simulink library "Kitchen_Lib"  (R2023a)
settings: Solver=VariableStepAuto  StartTime=0.0  StopTime=10.0  RelTol=1e-3  EnableMultiTasking=on
undefined symbols (not defined in the file): Kitc_BusTyp_P, Kitc_BusTypSkyr_C, Kitc_ColrLedColrls_C, Kitc_ColrLedGrn_C, Kitc_ColrLedRed_C, Kitc_ColrLedYlw_C, Kitc_StDgnWtrTank_C, Kitc_StElecPlugScktOffByClmp50_P, Kitc_StsDlyBlink_C, Kitc_StsErrBlink_C, Kitc_StsFctAcvn_P, Kitc_StsInfoBlink_C, Kitc_StsKitchnOffAutoIgOff_P, Kitc_StsKitchnOffBySwt_P, Kitc_StsKitchnOffDoorLockd_P, Kitc_StsKitchnOffIgOff_P, Kitc_StsKitchnOffUv_P, Kitc_StsKitchnOnBySwt_P, Kitc_StsKitchnOnNVM_P, Kitc_StsLedOff_C, Kitc_StsLedOn_C, Kitc_StsLrgCnsAcv_P, Kitc_StTrfrAnSwtInstd_P, Kitc_StTrfrSwtInstd_P, Kitc_TiKitcRefgtrOffDly_P, Kitc_ULowrThdBat_C, Kitc_UUpprThdBat_C, Kitc_ValFalse_C, Kitc_ValPwmFreq2_C, Kitc_ValPwmFreq_C, Kitc_ValTrue_C
libraries: MAN_Library x50, E2E_Lib x3
(part 2 of 13)

== system Kitchen_Lib/Kitchen/100ms/Kitchn/Subsystem1/Subsystem1 ==
  Kitc_StsHostsCallAcv : Inport
  BOOLEAN_TO_UINT8_Signals : Subsystem  AncestorBlock=E2E_Lib/BOOLEAN_TO_UINT8_Signals
  Logical Operator1 : Logic  Operator=NOT  AllPortsSameDT=off  OutDataTypeStr=boolean
  LogicalOperator25 : Logic  AllPortsSameDT=off  OutDataTypeStr=boolean
  Terminator : Terminator
  Terminator1 : Terminator
  Kitc_StsHostsCallAcv_E2E : Outport
  wires:
  Logical Operator1/1 -> LogicalOperator25/1
  BOOLEAN_TO_UINT8_Signals/3(Error) -> Terminator/1
  BOOLEAN_TO_UINT8_Signals/1(SignalOff) -> Logical Operator1/1
  BOOLEAN_TO_UINT8_Signals/4(NotInstalled_NotAvailable) -> Terminator1/1
  Kitc_StsHostsCallAcv/1 -> BOOLEAN_TO_UINT8_Signals/1(BOOLEAN_TO_UINT8_SignalIn)
  BOOLEAN_TO_UINT8_Signals/2(Signal|On) -> LogicalOperator25/2
  LogicalOperator25/1 -> Kitc_StsHostsCallAcv_E2E/1

== system Kitchen_Lib/Kitchen/100ms/Kitchn/Subsystem1/Subsystem10 ==
  GW_W_output : Inport
  Terminator40 : Terminator
  Terminator41 : Terminator
  UINT8_Signal : Subsystem  AncestorBlock=E2E_Lib/UINT8_Signal
  wires:
  UINT8_Signal/1(Error) -> Terminator40/1
  GW_W_output/1 -> UINT8_Signal/1(UINT8_SignalIn)
  UINT8_Signal/2(NotInstalled_NotAvailable) -> Terminator41/1

== system Kitchen_Lib/Kitchen/100ms/Kitchn/Subsystem1/Subsystem11 ==
  GW_BusTyp : Inport
  Terminator40 : Terminator
  Terminator41 : Terminator
  UINT8_Signal : Subsystem  AncestorBlock=E2E_Lib/UINT8_Signal
  wires:
  UINT8_Signal/2(NotInstalled_NotAvailable) -> Terminator41/1
  GW_BusTyp/1 -> UINT8_Signal/1(UINT8_SignalIn)
  UINT8_Signal/1(Error) -> Terminator40/1

== system Kitchen_Lib/Kitchen/100ms/Kitchn/Subsystem1/Subsystem12 ==
  GW_SpdGrtr3 : Inport
  BOOLEAN_TO_UINT8_Signals : Subsystem  AncestorBlock=E2E_Lib/BOOLEAN_TO_UINT8_Signals
  Logical Operator : Logic  AllPortsSameDT=off  OutDataTypeStr=boolean
  Logical Operator1 : Logic  Operator=NOT  AllPortsSameDT=off  OutDataTypeStr=boolean
  Terminator : Terminator
  Terminator1 : Terminator
  GW_SpdGrtr3_E2E : Outport
  wires:
  BOOLEAN_TO_UINT8_Signals/2(Signal|On) -> Logical Operator/2
  BOOLEAN_TO_UINT8_Signals/4(NotInstalled_NotAvailable) -> Terminator1/1
  BOOLEAN_TO_UINT8_Signals/3(Error) -> Terminator/1
  Logical Operator1/1 -> Logical Operator/1
  GW_SpdGrtr3/1 -> BOOLEAN_TO_UINT8_Signals/1(BOOLEAN_TO_UINT8_SignalIn)
  Logical Operator/1 -> GW_SpdGrtr3_E2E/1
  BOOLEAN_TO_UINT8_Signals/1(SignalOff) -> Logical Operator1/1

== system Kitchen_Lib/Kitchen/100ms/Kitchn/Subsystem1/Subsystem13 ==
  DBF_StsDoor1Open : Inport
  BOOLEAN_TO_UINT8_Signals : Subsystem  AncestorBlock=E2E_Lib/BOOLEAN_TO_UINT8_Signals
  Logical Operator1 : Logic  Operator=NOT  AllPortsSameDT=off  OutDataTypeStr=boolean
  LogicalOperator25 : Logic  AllPortsSameDT=off  OutDataTypeStr=boolean
  Terminator : Terminator
  Terminator1 : Terminator
  DBF_StsDoor1Open_E2E : Outport
  wires:
  BOOLEAN_TO_UINT8_Signals/3(Error) -> Terminator/1
  BOOLEAN_TO_UINT8_Signals/1(SignalOff) -> Logical Operator1/1
  BOOLEAN_TO_UINT8_Signals/4(NotInstalled_NotAvailable) -> Terminator1/1
  DBF_StsDoor1Open/1 -> BOOLEAN_TO_UINT8_Signals/1(BOOLEAN_TO_UINT8_SignalIn)
  BOOLEAN_TO_UINT8_Signals/2(Signal|On) -> LogicalOperator25/2
  LogicalOperator25/1 -> DBF_StsDoor1Open_E2E/1
  Logical Operator1/1 -> LogicalOperator25/1

== system Kitchen_Lib/Kitchen/100ms/Kitchn/Subsystem1/Subsystem14 ==
  Toi_ToiInstlldInfo : Inport
  BOOLEAN_TO_UINT8_Signals : Subsystem  AncestorBlock=E2E_Lib/BOOLEAN_TO_UINT8_Signals
  Logical Operator1 : Logic  Operator=NOT  AllPortsSameDT=off  OutDataTypeStr=boolean
  LogicalOperator25 : Logic  AllPortsSameDT=off  OutDataTypeStr=boolean
  Terminator : Terminator
  Terminator1 : Terminator
  Toi_ToiInstlldInfo_E2E : Outport
  wires:
  Logical Operator1/1 -> LogicalOperator25/1
  LogicalOperator25/1 -> Toi_ToiInstlldInfo_E2E/1
  BOOLEAN_TO_UINT8_Signals/2(Signal|On) -> LogicalOperator25/2
  Toi_ToiInstlldInfo/1 -> BOOLEAN_TO_UINT8_Signals/1(BOOLEAN_TO_UINT8_SignalIn)
  BOOLEAN_TO_UINT8_Signals/4(NotInstalled_NotAvailable) -> Terminator1/1
  BOOLEAN_TO_UINT8_Signals/1(SignalOff) -> Logical Operator1/1
  BOOLEAN_TO_UINT8_Signals/3(Error) -> Terminator/1

== system Kitchen_Lib/Kitchen/100ms/Kitchn/Subsystem1/Subsystem15 ==
  Kitc_StDemoBd : Inport
  BOOLEAN_TO_UINT8_Signals : Subsystem  AncestorBlock=E2E_Lib/BOOLEAN_TO_UINT8_Signals
  Logical Operator1 : Logic  Operator=NOT  AllPortsSameDT=off  OutDataTypeStr=boolean
  LogicalOperator25 : Logic  AllPortsSameDT=off  OutDataTypeStr=boolean
  Terminator : Terminator
  Terminator1 : Terminator
  Kitc_StDemoBd_E2E : Outport
  wires:
  Logical Operator1/1 -> LogicalOperator25/1
  BOOLEAN_TO_UINT8_Signals/3(Error) -> Terminator/1
  BOOLEAN_TO_UINT8_Signals/1(SignalOff) -> Logical Operator1/1
  BOOLEAN_TO_UINT8_Signals/4(NotInstalled_NotAvailable) -> Terminator1/1
  Kitc_StDemoBd/1 -> BOOLEAN_TO_UINT8_Signals/1(BOOLEAN_TO_UINT8_SignalIn)
  BOOLEAN_TO_UINT8_Signals/2(Signal|On) -> LogicalOperator25/2
  LogicalOperator25/1 -> Kitc_StDemoBd_E2E/1

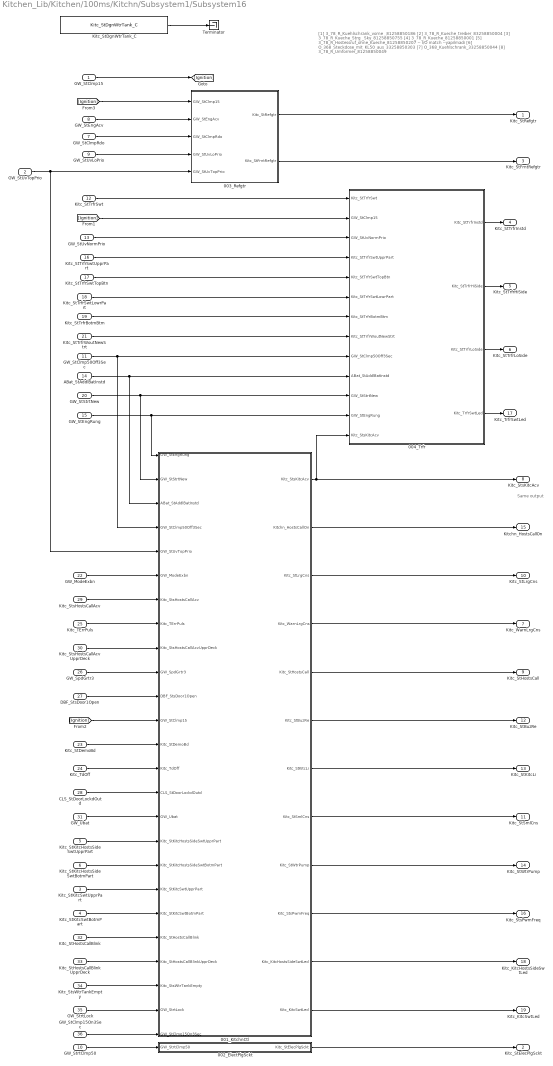
== system Kitchen_Lib/Kitchen/100ms/Kitchn/Subsystem1/Subsystem16 ==
  note: Same output
  note: [1] 3_78_R_Kuehlschrank_vorne _81258850186
      | [2] 3_78_R_Kueche_treiber_83258850004
      | [3] 3_78_R_Kueche_Strg _Sky_81258850755
      | [4] 3_78_R_Kueche_81258850001
      | [5] 3_78_R_Hostessruf_ohne_Kueche_81258850207 -- I/O match --yapilmadi
      | [6] O_368_Steckdose_mit_KL50_aus_33258850303
      | [7] O_368_Kuehlschrank_33258850044
      | [8] 3_78_R_Umformer_81258850049
  GW_StClmp15 : Inport
  "GW_StUvTopPrio " : Inport  Port=2
  Kitc_StKitcSwtUpprPart : Inport  Port=3
  Kitc_StKitcSwtBotmPart : Inport  Port=4
  Kitc_StKitcHostsSideSwtUpprPart : Inport  Port=5
  Kitc_StKitcHostsSideSwtBotmPart : Inport  Port=6
  GW_StClmpRdo : Inport  Port=7
  "GW_StEngAcv " : Inport  Port=8
  "GW_StUvLoPrio " : Inport  Port=9
  "GW_StrtClmp50 " : Inport  Port=10
  "GW_StClmp50Off3Sec " : Inport  Port=11
  "Kitc_StTrfrSwt " : Inport  Port=12
  "GW_StUvNormPrio " : Inport  Port=13
  ABat_StAddlBatInstd : Inport  Port=14
  GW_StEngRung : Inport  Port=15
  Kitc_StTrfrSwtUpprPart : Inport  Port=16
  Kitc_StTrfrSwtTopBtn : Inport  Port=17
  Kitc_StTrfrSwtLowrPart : Inport  Port=18
  Kitc_StTrfrBotmBtm : Inport  Port=19
  "GW_StStrtNew " : Inport  Port=20
  Kitc_StTrfrWoutNewStrt : Inport  Port=21
  "GW_ModeExbn " : Inport  Port=22
  Kitc_StDemoBd : Inport  Port=23
  Kitc_TdOff : Inport  Port=24
  Kitc_TErrPuls : Inport  Port=25
  GW_SpdGrtr3 : Inport  Port=26
  DBF_StsDoor1Open : Inport  Port=27
  CLS_StDoorLockdOutd : Inport  Port=28
  Kitc_StsHostsCallAcv : Inport  Port=29
  Kitc_StsHostsCallAcvUpprDeck : Inport  Port=30
  "GW_Ubat " : Inport  Port=31
  Kitc_StHostsCallBlink : Inport  Port=32
  Kitc_StHostsCallBlinkUpprDeck : Inport  Port=33
  Kitc_StsWtrTankEmpty : Inport  Port=34
  "GW_StrtLock " : Inport  Port=35
  "GW_StClmp15On3Sec " : Inport  Port=36
  001_KitchnCtl : Subsystem
  002_ElectPlgSckt : Subsystem
  003_Refgtr : Subsystem
  004_Trfr : Subsystem
  Kitc_StDgnWtrTank_C : Constant  Value=Kitc_StDgnWtrTank_C
  Terminator : Terminator
  Kitc_StRefgtr : Outport
  Kitc_StElecPlgSckt : Outport  Port=2
  Kitc_StFrntRefgtr : Outport  Port=3
  Kitc_StTrfrInstd : Outport  Port=4
  Kitc_StTrfrHiSide : Outport  Port=5
  Kitc_StTrfrLoSide : Outport  Port=6
  Kitc_WarnLrgCns : Outport  Port=7
  Kitc_StsKitcAcv : Outport  Port=8
  Kitc_StHostsCall : Outport  Port=9
  Kitc_StLrgCns : Outport  Port=10
  Kitc_StSmlCns : Outport  Port=11
  Kitc_StBuzRe : Outport  Port=12
  Kitc_StKitcLi : Outport  Port=13
  Kitc_StWtrPump : Outport  Port=14
  Kitchn_HostsCallOn : Outport  Port=15
  Kitc_StsPwmFreq : Outport  Port=16
  Kitc_TrfrSwtLed : Outport  Port=17
  Kitc_KitcHostsSideSwtLed : Outport  Port=18
  Kitc_KitcSwtLed : Outport  Port=19
  wires:
  "GW_StUvTopPrio "/1 -> 001_KitchnCtl/5("GW_StUvTopPrio "), 003_Refgtr/5("GW_StUvTopPrio ")
  Kitc_StKitcSwtUpprPart/1 -> 001_KitchnCtl/19(Kitc_StKitcSwtUpprPart)
  "GW_StEngAcv "/1 -> 003_Refgtr/2("GW_StEngAcv ")
  Kitc_StKitcSwtBotmPart/1 -> 001_KitchnCtl/20(Kitc_StKitcSwtBotmPart)
  "Kitc_StTrfrSwt "/1 -> 004_Trfr/1("Kitc_StTrfrSwt ")
  "GW_StClmp50Off3Sec "/1 -> 001_KitchnCtl/4("GW_StClmp50Off3Sec "), 004_Trfr/9("GW_StClmp50Off3Sec ")
  001_KitchnCtl/1(Kitc_StsKitcAcv) -> 004_Trfr/13(Kitc_StsKitcAcv), Kitc_StsKitcAcv/1
  "GW_StUvNormPrio "/1 -> 004_Trfr/3("GW_StUvNormPrio ")
  Kitc_StKitcHostsSideSwtBotmPart/1 -> 001_KitchnCtl/18(Kitc_StKitcHostsSideSwtBotmPart)
  "GW_StUvLoPrio "/1 -> 003_Refgtr/4("GW_StUvLoPrio ")
  "GW_StrtClmp50 "/1 -> 002_ElectPlgSckt/1("GW_StrtClmp50 ")
  Kitc_StKitcHostsSideSwtUpprPart/1 -> 001_KitchnCtl/17(Kitc_StKitcHostsSideSwtUpprPart)
  [Ignition] -> 003_Refgtr/1(GW_StClmp15)
  GW_StClmpRdo/1 -> 003_Refgtr/3(GW_StClmpRdo)
  Kitc_StsHostsCallAcv/1 -> 001_KitchnCtl/7(Kitc_StsHostsCallAcv)
  ABat_StAddlBatInstd/1 -> 001_KitchnCtl/3(ABat_StAddlBatInstd), 004_Trfr/10(ABat_StAddlBatInstd)
  Kitc_StTrfrSwtUpprPart/1 -> 004_Trfr/4(Kitc_StTrfrSwtUpprPart)
  GW_StClmp15/1 -> [Ignition]
  GW_StEngRung/1 -> 001_KitchnCtl/1(GW_StEngRung), 004_Trfr/12(GW_StEngRung)
  Kitc_TdOff/1 -> 001_KitchnCtl/14(Kitc_TdOff)
  Kitc_TErrPuls/1 -> 001_KitchnCtl/8(Kitc_TErrPuls)
  Kitc_StsHostsCallAcvUpprDeck/1 -> 001_KitchnCtl/9(Kitc_StsHostsCallAcvUpprDeck)
  Kitc_StTrfrSwtTopBtn/1 -> 004_Trfr/5(Kitc_StTrfrSwtTopBtn)
  "GW_StStrtNew "/1 -> 001_KitchnCtl/2("GW_StStrtNew "), 004_Trfr/11("GW_StStrtNew ")
  "GW_ModeExbn "/1 -> 001_KitchnCtl/6("GW_ModeExbn ")
  [Ignition] -> 004_Trfr/2(GW_StClmp15)
  [Ignition] -> 001_KitchnCtl/12(GW_StClmp15)
  GW_SpdGrtr3/1 -> 001_KitchnCtl/10(GW_SpdGrtr3)
  Kitc_StTrfrWoutNewStrt/1 -> 004_Trfr/8(Kitc_StTrfrWoutNewStrt)
  Kitc_StTrfrSwtLowrPart/1 -> 004_Trfr/6(Kitc_StTrfrSwtLowrPart)
  Kitc_StDemoBd/1 -> 001_KitchnCtl/13(Kitc_StDemoBd)
  CLS_StDoorLockdOutd/1 -> 001_KitchnCtl/15(CLS_StDoorLockdOutd)
  DBF_StsDoor1Open/1 -> 001_KitchnCtl/11(DBF_StsDoor1Open)
  Kitc_StTrfrBotmBtm/1 -> 004_Trfr/7(Kitc_StTrfrBotmBtm)
  "GW_Ubat "/1 -> 001_KitchnCtl/16("GW_Ubat ")
  Kitc_StsWtrTankEmpty/1 -> 001_KitchnCtl/23(Kitc_StsWtrTankEmpty)
  Kitc_StHostsCallBlink/1 -> 001_KitchnCtl/21(Kitc_StHostsCallBlink)
  "GW_StClmp15On3Sec "/1 -> 001_KitchnCtl/25("GW_StClmp15On3Sec ")
  "GW_StrtLock "/1 -> 001_KitchnCtl/24("GW_StrtLock ")
  Kitc_StHostsCallBlinkUpprDeck/1 -> 001_KitchnCtl/22(Kitc_StHostsCallBlinkUpprDeck)
  002_ElectPlgSckt/1(Kitc_StElecPlgSckt) -> Kitc_StElecPlgSckt/1
  001_KitchnCtl/8(Kitc_StSmlCns) -> Kitc_StSmlCns/1
  001_KitchnCtl/7(Kitc_StKitcLi) -> Kitc_StKitcLi/1
  001_KitchnCtl/6(Kitc_StBuzRe) -> Kitc_StBuzRe/1
  001_KitchnCtl/5(Kitc_StHostsCall) -> Kitc_StHostsCall/1
  001_KitchnCtl/4(Kitc_WarnLrgCns) -> Kitc_WarnLrgCns/1
  001_KitchnCtl/3(Kitc_StLrgCns) -> Kitc_StLrgCns/1
  004_Trfr/3(Kitc_StTrfrLoSide) -> Kitc_StTrfrLoSide/1
  004_Trfr/2(Kitc_StTrfrHiSide) -> Kitc_StTrfrHiSide/1
  004_Trfr/1(Kitc_StTrfrInstd) -> Kitc_StTrfrInstd/1
  003_Refgtr/2("Kitc_StFrntRefgtr ") -> Kitc_StFrntRefgtr/1
  003_Refgtr/1(Kitc_StRefgtr) -> Kitc_StRefgtr/1
  001_KitchnCtl/9(Kitc_StWtrPump) -> Kitc_StWtrPump/1
  001_KitchnCtl/2(Kitchn_HostsCallOn) -> Kitchn_HostsCallOn/1
  001_KitchnCtl/10(Kitc_StsPwmFreq) -> Kitc_StsPwmFreq/1
  Kitc_StDgnWtrTank_C/1 -> Terminator/1
  004_Trfr/4(Kitc_TrfrSwtLed) -> Kitc_TrfrSwtLed/1
  001_KitchnCtl/11(Kitc_KitcHostsSideSwtLed) -> Kitc_KitcHostsSideSwtLed/1
  001_KitchnCtl/12(Kitc_KitcSwtLed) -> Kitc_KitcSwtLed/1

== system Kitchen_Lib/Kitchen/100ms/Kitchn/Subsystem1/Subsystem17 ==
  Kitc_TdOff_E2E : Inport
  Terminator40 : Terminator
  Terminator41 : Terminator
  UINT32_Signal : Subsystem  AncestorBlock=E2E_Lib/UINT32_Signal
  wires:
  UINT32_Signal/1(Error) -> Terminator40/1
  UINT32_Signal/2(NotInstalled_NotAvailable) -> Terminator41/1
  Kitc_TdOff_E2E/1 -> UINT32_Signal/1(UINT32_SignalIn)

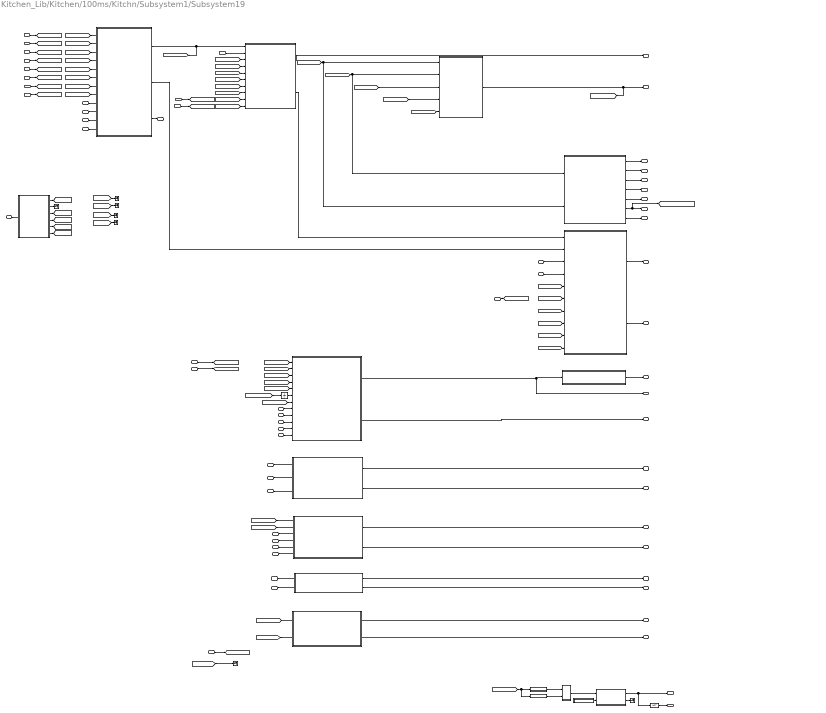
== system Kitchen_Lib/Kitchen/100ms/Kitchn/Subsystem1/Subsystem19 ==
  note: APPLICATION LOGIC
  note: OUTPUTS
  note: Skyliner
  note: EIO_B26 1Pin5
      | DigOut
      |
      | Kitc_StBuzRe
      | The pin of the call bell is given as a socket.
      | It is not connected to a serial or SA location on the device
      |
      | EIO_B26 4Pin22
      | DigOut
      | Kitc_StsKitcAcv
      | Kitchen activation signal.
      |
      | EIO_B26 1Pin2
      | PWMOut
      |
      | Kitc_StLrgCns
      |
      | It is the trigger pin that serves to activate the kitchen. When the button located in the fap section is pressed, the kitchen system is activated, and these pins are the trigger pins.
      |
      | EIO_B26 5Pin6
      | PWMOut
      |
      | Kitc_StSmlCns
      | There are two mode.
      | -When car is moving Large consumption mode is activated.
      | -When car is stopping Small consumption mode is activated.
      |
      | EIO_B26 5Pin7
      | DigOut
      |
      | Kitc_StTrfr
      | Kitchen power supply electrical plag.
      |
      | EIO_B26 3Pin2
      | DigInp
      |
      | Kitc_EidWtrTankEmpty
      | It reports the water level in the tank and sends a warning to the driver when the water runs out in the clean water
      |
      | EIO_B26 1Pin8
      | DigOut
      |
      | Kitc_StRefgtr
      | It is used for the refrigerator in cases where the refrigerator comes in the toilet
      |
      | EIO_B26 3Pin41
      | PWMOut
      | Kitc_StHostsCall
      | It is used for the hostess call Skyliner
  note: Shutdown Request
  Kitc_StKitcSwtUpprPart : Inport
  Kitc_StKitcHostsSideSwtUpprPart : Inport  Port=2
  Kitc_StKitcHostsSideSwtBotmPart : Inport  Port=3
  GW_StBttrySupplyVltMVBSWOn : Inport  Port=4
  "GW_ModeExbn " : Inport  Port=5
  GW_SpdGrtr3 : Inport  Port=6
  CLS_StDoorLockdOutd : Inport  Port=7
  "GW_StStrtNew " : Inport  Port=8
  GW_StUvTopPrio : Inport  Port=9
  GW_StClmp15 : Inport  Port=10
  DBF_StsDoor1Open : Inport  Port=11
  GW_StEngRung : Inport  Port=12
  ABat_StAddlBatInstd : Inport  Port=13
  Kitc_StsHostsCallAcv : Inport  Port=14
  "GW_StClmp50Off3Sec " : Inport  Port=15
  "GW_StUvNormPrio " : Inport  Port=16
  Kitc_StHostsCallBlink : Inport  Port=17
  Kitc_StHostsCallBlinkUpprDeck : Inport  Port=18
  Kitc_StsWtrTankEmpty : Inport  Port=19
  "GW_StrtLock " : Inport  Port=20
  "GW_StClmp15On3Sec " : Inport  Port=21
  Kitc_StsHostsCallAcvUpprDeck : Inport  Port=22
  Kitc_TErrPuls : Inport  Port=23
  Kitc_StTrfrSwtUpprPart : Inport  Port=24
  Kitc_StTrfrSwtTopBtn : Inport  Port=25
  Kitc_StTrfrBotmBtm : Inport  Port=26
  Kitc_StTrfrWoutNewStrt : Inport  Port=27
  "Kitc_StTrfrSwt " : Inport  Port=28
  "GW_StEngAcv " : Inport  Port=29
  GW_StClmpRdo : Inport  Port=30
  "GW_StUvLoPrio " : Inport  Port=31
  Toi_ToiInstlldInfo : Inport  Port=32
  Kitc_StDemoBd : Inport  Port=33
  Kitc_TdOff : Inport  Port=34
  GW_W_output : Inport  Port=35
  GW_BusTyp : Inport  Port=36
  003_TrfrSwtLed : Subsystem
  BusTypeSelection : Subsystem  AncestorBlock=MAN_Library/BusTypeSelection
  Cluster_Message : Subsystem
  FallingEdgeDetection : Subsystem  AncestorBlock=MAN_Library/FallingEdgeDetection
  KSW_Battery : Subsystem
  KitchenActive : Subsystem
  KitchenDriver : Subsystem
  KitchenEnable : Subsystem
  KitchenSwtLed : Subsystem
  Logical Operator : Logic  Operator=NOT  AllPortsSameDT=off  OutDataTypeStr=boolean
  PWMOutput : Subsystem
  Refgtr : Subsystem
  RisingEdgeDetection : Subsystem  AncestorBlock=MAN_Library/RisingEdgeDetection
  SR : Subsystem  AncestorBlock=MAN_Library/SR
  Terminator{,1..6} (7 alike) : Terminator
  TimeConstant : Subsystem  AncestorBlock=MAN_Library/TimeConstant  mask{hours=0, minutes=30, seconds=0, miliseconds=0}
      mask prompts: hours "Hour"
      mask DialogControl TimeConstant Prompt: Time Constant
      mask Display:
      | timeDraw = 'Time#';
      | if( hours == 0 && minutes == 0 && seconds == 0 && miliseconds == 0)
      |     timeDraw = strcat(timeDraw,'0secs'),
      | else
      |     if( hours ~= 0)
      |         timeDraw = strcat(timeDraw,num2str(hours),'hours');
      |     end
      |     if( minutes ~= 0)
      |         timeDraw = strcat(timeDraw,num2str(minutes),'min');
      |     end
      |     if( seconds ~= 0)
      |         timeDraw = strcat(timeDraw,num2str(seconds),'sec');
      |     end
      |     if( miliseconds ~= 0)
      |         timeDraw = strcat(timeDraw,num2str(miliseconds),'ms');
      |     end
      | end
      | fprintf(timeDraw);
  TimePulse : Subsystem  AncestorBlock=MAN_Library/TimePulse  mask(Time Pulse){CycleTime=Cycle Time: 10 Ms}
      mask prompts: CycleTime "Select the Cycle Time:"
      mask help:
      | This is a PULSE GENERATOR producing a pulse, if there is a positive-going edge at input IN. The length of the pulse which should be generated is defined by input PT. After the occurrence of the positive edge output Q is set to HIGH for the period of time defined in PT. Output ET counts the time - beginning with the occurrence of the positive edge - until the value set at PT has been reached. The value in ET is kept as long as the input IN has the state of HIGH.
      |
      | IN : Timer starting bit
      | PT : Preset time of timer
      | Q  : Time pulse flag
      | ET : Current value of timer
      mask TypeOptions CycleTime: Cycle Time: 1 Ms | Cycle Time: 10 Ms | Cycle Time: 100 Ms | Cycle Time: 1000 Ms
      mask Display:
      | disp('{\bf\fontsize{18}Time Pulse}', 'texmode','on');
      | 
      | port_label('input', 1,'IN');
      | port_label('input', 2,'PT');
      | port_label('output',1,'Q');
      | port_label('output',2,'ET');
  Trfr : Subsystem
  Unit Delay : UnitDelay  SampleTime=-1  HasFrameUpgradeWarning=on
  WaterTankEmptyDiagnostic : Subsystem
  Kitc_StsKitcAcv : Outport
  Kitc_StBuzRe : Outport  Port=2
  Kitc_StLrgCns : Outport  Port=3
  Kitc_StSmlCns : Outport  Port=4
  Kitc_StsPwmFreq : Outport  Port=5
  Kitc_StTrfr : Outport  Port=6
  Kitc_TrfrSwtLed : Outport  Port=7
  Kitc_KitcHostsSideSwtLed : Outport  Port=8
  Kitc_KitcSwtLed : Outport  Port=9
  Kitc_EidWtrTankEmpty : Outport  Port=10
  Kitc_StRefgtr : Outport  Port=11
  Kitc_StHostsCall : Outport  Port=12
  Kitchn_StAcvCode : Outport  Port=13
  Kitc_StTrfrInstd : Outport  Port=14
  "Kitc_StFrntRefgtr " : Outport  Port=15
  Kitc_PwmHostsCall : Outport  Port=16
  Kitc_KtchnLowBttryNotRlsd : Outport  Port=17
  Kitc_StsPwmFreq2 : Outport  Port=18
  Kitc_AcvSkyliner : Outport  Port=19
  Kitc_ShtdwnReqPermsn : Outport  Port=20
  Kitc_ShtdwnReqBlck : Outport  Port=21
  Kitc_KitchenReleased : Outport  Port=22
  Kitc_KitchenNotReleased : Outport  Port=23
  Kitch_dispWtrTnkLvlWrng : Outport  Port=24
  Kitch_dispKitchenPssngrReqAcv : Outport  Port=25
  wires:
  Cluster_Message/2(Kitch_dispKitchenPssngrReqAcv) -> Kitch_dispKitchenPssngrReqAcv/1
  WaterTankEmptyDiagnostic/2(Kitch_dispWtrTnkLvlWrng) -> Kitch_dispWtrTnkLvlWrng/1
  [SleepMode] -> Terminator6/1
  [Kitc_KitchenReleased] -> Cluster_Message/2(Kitc_KitchenReleased)
  PWMOutput/7(Kitc_KitchenNotReleased) -> Kitc_KitchenNotReleased/1
  PWMOutput/6(Kitc_KitchenReleased) -> Kitc_KitchenReleased/1, [Kitc_KitchenReleased]
  TimePulse/2(TimePulseExpiredTime) -> Terminator5/1
  TimePulse/1(TimePulseFlag) -> Kitc_ShtdwnReqPermsn/1, Logical Operator/1
  TimeConstant/1(time) -> TimePulse/2(TimePulseDuration)
  SR/1(Q) -> TimePulse/1(TimePulseEnable)
  [GW_StClmp15] -> FallingEdgeDetection/1(CLK), RisingEdgeDetection/1(CLK)
  Logical Operator/1 -> Kitc_ShtdwnReqBlck/1
  RisingEdgeDetection/1(Q) -> SR/2(R)
  FallingEdgeDetection/1(Q) -> SR/1(S)
  PWMOutput/5(Kitc_AcvSkyliner) -> Kitc_AcvSkyliner/1
  BusTypeSelection/2(BusTypCityStep2) -> Terminator4/1
  BusTypeSelection/6(BusTypElec) -> [BusTypElec]
  BusTypeSelection/5(BusTypSky) -> [BusTypSky]
  BusTypeSelection/4(BusTypIntercity) -> [BusTypIntercity]
  BusTypeSelection/3(BusTypCoach) -> [BusTypCoach]
  PWMOutput/4(Kitc_StsPwmFreq2) -> Kitc_StsPwmFreq2/1
  [BusTypSky] -> KitchenSwtLed/10(Kitc_BusTypSkyr)
  [BusTypSky] -> KitchenActive/5(Kitc_BusTypSkyr)
  [BusTypIntercity] -> Terminator3/1
  [BusTypCoach] -> Terminator2/1
  [BusTypElec] -> Terminator1/1
  GW_BusTyp/1 -> BusTypeSelection/1(GW_BusTyp)
  [BusTypCity] -> Terminator/1
  BusTypeSelection/1(BusTypCityStep1) -> [BusTypCity]
  [GW_StUvTopPrio] -> Cluster_Message/1(GW_StUvTopPrio)
  Cluster_Message/1(Kitc_KtchnLowBttryNotRlsd) -> Kitc_KtchnLowBttryNotRlsd/1
  GW_W_output/1 -> [SleepMode]
  KitchenDriver/2(Kitc_PwmHostsCall) -> Kitc_PwmHostsCall/1
  Refgtr/2("Kitc_StFrntRefgtr ") -> "Kitc_StFrntRefgtr "/1
  Trfr/2(Kitc_StTrfrInstd) -> Kitc_StTrfrInstd/1
  Kitc_StKitcHostsSideSwtBotmPart/1 -> KitchenEnable/12(Kitc_StKitcHostsSideSwtBotmPart)
  Kitc_StKitcHostsSideSwtUpprPart/1 -> KitchenEnable/11(Kitc_StKitcHostsSideSwtUpprPart)
  Kitc_TdOff/1 -> KitchenEnable/10(Kitc_TdOff)
  Kitc_StDemoBd/1 -> KitchenEnable/9(Kitc_StDemoBd)
  Toi_ToiInstlldInfo/1 -> Refgtr/6(Toi_ToiInstlldInfo)
  "GW_StUvLoPrio "/1 -> Refgtr/5("GW_StUvLoPrio ")
  GW_StClmpRdo/1 -> Refgtr/4(GW_StClmpRdo)
  "GW_StEngAcv "/1 -> Refgtr/3("GW_StEngAcv ")
  [GW_StUvTopPrio] -> Refgtr/2("GW_StUvTopPrio ")
  KitchenEnable/3(Kitchn_StAcvCode) -> Kitchn_StAcvCode/1
  "Kitc_StTrfrSwt "/1 -> Trfr/8("Kitc_StTrfrSwt ")
  Unit Delay/1 -> Trfr/6(Kitc_StsKitcAcv)
  [GW_StClmp15] -> Trfr/5(GW_StClmp15)
  [GW_StEngRung] -> Trfr/4(GW_StEngRung)
  [ABat_StAddlBatInstd] -> Trfr/3(ABat_StAddlBatInstd)
  [GW_StUvNormPrio] -> Trfr/2("GW_StUvNormPrio ")
  [GW_StClmp50Off3Sec] -> Trfr/1("GW_StClmp50Off3Sec ")
  Kitc_StTrfrWoutNewStrt/1 -> Trfr/12(Kitc_StTrfrWoutNewStrt)
  [GW_StStrtNew] -> Trfr/7("GW_StStrtNew ")
  Kitc_StTrfrBotmBtm/1 -> Trfr/11(Kitc_StTrfrBotmBtm)
  Kitc_StTrfrSwtTopBtn/1 -> Trfr/10(Kitc_StTrfrSwtTopBtn)
  Kitc_StTrfrSwtUpprPart/1 -> Trfr/9(Kitc_StTrfrSwtUpprPart)
  003_TrfrSwtLed/1(Kitc_TrfrSwtLed) -> Kitc_TrfrSwtLed/1
  "GW_StUvNormPrio "/1 -> [GW_StUvNormPrio]
  KitchenEnable/2(HostsSideBtnErr) -> KitchenSwtLed/2(HostsSideBtnErr)
  [DBF_StsDoor1Open] -> KitchenEnable/8(DBF_StsDoor1Open)
  [GW_SpdGrtr3] -> KitchenEnable/7(GW_SpdGrtr3)
  GW_StEngRung/1 -> [GW_StEngRung]
  KitchenDriver/1(Kitc_StHostsCall) -> Kitc_StHostsCall/1
  Refgtr/1(Kitc_StRefgtr) -> Kitc_StRefgtr/1
  WaterTankEmptyDiagnostic/1(Kitc_EidWtrTankEmpty) -> Kitc_EidWtrTankEmpty/1
  Kitc_TErrPuls/1 -> KitchenSwtLed/4(Kitc_TErrPuls)
  Kitc_StsHostsCallAcvUpprDeck/1 -> KitchenSwtLed/3(Kitc_StsHostsCallAcvUpprDeck)
  [GW_StUvTopPrio] -> KitchenSwtLed/9("GW_StUvTopPrio ")
  [Kitc_StKitcSwtUpprPart] -> KitchenSwtLed/5(Kitc_StKitcSwtUpprPart)
  [Kitc_StsHostsCallAcv] -> KitchenSwtLed/6(Kitc_StsHostsCallAcv)
  [GW_ModeExbn] -> KitchenSwtLed/8("GW_ModeExbn ")
  [Kitchn_On] -> KitchenSwtLed/7(Kitchn_On)
  KSW_Battery/2(Kitc_WarnLrgCns) -> KitchenSwtLed/1(Kitc_WarnLrgCns)
  KitchenSwtLed/2(Kitc_KitcSwtLed) -> Kitc_KitcSwtLed/1
  KitchenSwtLed/1(Kitc_KitcHostsSideSwtLed) -> Kitc_KitcHostsSideSwtLed/1
  "GW_StClmp15On3Sec "/1 -> WaterTankEmptyDiagnostic/3("GW_StClmp15On3Sec ")
  "GW_StrtLock "/1 -> WaterTankEmptyDiagnostic/2("GW_StrtLock ")
  Kitc_StsWtrTankEmpty/1 -> WaterTankEmptyDiagnostic/1(Kitc_StsWtrTankEmpty)
  KitchenActive/1(Kitc_StsKitcAcv) -> [Kitc_StsKitcAcv], Kitc_StsKitcAcv/1
  [GW_StEngRung] -> KitchenActive/4(GW_StEngRung)
  [ABat_StAddlBatInstd] -> KitchenActive/3(ABat_StAddlBatInstd)
  [Kitchn_On] -> PWMOutput/2(KitchnOn), KitchenActive/1(Kitchn_On)
  "GW_StClmp50Off3Sec "/1 -> [GW_StClmp50Off3Sec]
  [GW_StClmp50Off3Sec] -> KSW_Battery/6("GW_StClmp50Off3Sec ")
  [GW_StEngRung] -> KSW_Battery/9(GW_StEngRung)
  [ABat_StAddlBatInstd] -> KSW_Battery/10(ABat_StAddlBatInstd)
  ABat_StAddlBatInstd/1 -> [ABat_StAddlBatInstd]
  [GW_StClmp15] -> KitchenEnable/6(GW_StClmp15)
  [GW_StUvTopPrio] -> KitchenEnable/5("GW_StUvTopPrio ")
  [GW_ModeExbn] -> KitchenEnable/4("GW_ModeExbn ")
  [GW_StStrtNew] -> KitchenEnable/3("GW_StStrtNew ")
  [CLS_StDoorLockdOutd] -> KitchenEnable/2(CLS_StDoorLockdOutd)
  [Kitc_StKitcSwtUpprPart] -> KitchenEnable/1(Kitc_StKitcSwtUpprPart)
  Kitc_StKitcSwtUpprPart/1 -> [Kitc_StKitcSwtUpprPart]
  Kitc_StHostsCallBlinkUpprDeck/1 -> KitchenDriver/2(Kitc_StHostsCallBlinkUpprDeck)
  Kitc_StHostsCallBlink/1 -> KitchenDriver/1(Kitc_StHostsCallBlink)
  [Kitc_StsKitcAcv] -> Unit Delay/1
  [Kitc_StsHostsCallAcv] -> KSW_Battery/8(Kitc_StsHostsCallAcv)
  Kitc_StsHostsCallAcv/1 -> [Kitc_StsHostsCallAcv]
  [CLS_StDoorLockdOutd] -> KSW_Battery/7(CLS_StDoorLockdOutd)
  DBF_StsDoor1Open/1 -> [DBF_StsDoor1Open]
  GW_StClmp15/1 -> [GW_StClmp15]
  GW_StUvTopPrio/1 -> [GW_StUvTopPrio]
  "GW_StStrtNew "/1 -> [GW_StStrtNew]
  CLS_StDoorLockdOutd/1 -> [CLS_StDoorLockdOutd]
  [GW_StClmp15] -> Refgtr/1(GW_StClmp15)
  GW_SpdGrtr3/1 -> [GW_SpdGrtr3]
  "GW_ModeExbn "/1 -> [GW_ModeExbn]
  Trfr/1(Kitc_StTrfr) -> Kitc_StTrfr/1, 003_TrfrSwtLed/1(Fnc_On)
  PWMOutput/3(Kitc_StsPwmFreq) -> Kitc_StsPwmFreq/1
  PWMOutput/2(Kitc_StSmlCns) -> Kitc_StSmlCns/1
  PWMOutput/1(Kitc_StLrgCns) -> Kitc_StLrgCns/1
  [GW_StClmp15] -> PWMOutput/1(GW_StClmp15), KitchenActive/2(GW_StClmp15)
  KitchenEnable/1(Kitchn_On) -> KSW_Battery/1(Kitchn_On), [Kitchn_On]
  GW_StBttrySupplyVltMVBSWOn/1 -> KSW_Battery/2("GW_Ubat ")
  KSW_Battery/1(Kitc_StBuzRe) -> Kitc_StBuzRe/1
  [GW_StClmp15] -> KSW_Battery/3(GW_StClmp15)
  [GW_StUvTopPrio] -> KSW_Battery/4("GW_StUvTopPrio ")
  [GW_ModeExbn] -> KSW_Battery/5("GW_ModeExbn ")

== system Kitchen_Lib/Kitchen/100ms/Kitchn/Subsystem1/Subsystem2 ==
  ABat_StAddlBatInstd : Inport
  BOOLEAN_TO_UINT8_Signals : Subsystem  AncestorBlock=E2E_Lib/BOOLEAN_TO_UINT8_Signals
  Logical Operator1 : Logic  Operator=NOT  AllPortsSameDT=off  OutDataTypeStr=boolean
  LogicalOperator25 : Logic  AllPortsSameDT=off  OutDataTypeStr=boolean
  Terminator : Terminator
  Terminator1 : Terminator
  ABat_StAddlBatInstd_E2E : Outport
  wires:
  Logical Operator1/1 -> LogicalOperator25/1
  LogicalOperator25/1 -> ABat_StAddlBatInstd_E2E/1
  BOOLEAN_TO_UINT8_Signals/2(Signal|On) -> LogicalOperator25/2
  ABat_StAddlBatInstd/1 -> BOOLEAN_TO_UINT8_Signals/1(BOOLEAN_TO_UINT8_SignalIn)
  BOOLEAN_TO_UINT8_Signals/4(NotInstalled_NotAvailable) -> Terminator1/1
  BOOLEAN_TO_UINT8_Signals/1(SignalOff) -> Logical Operator1/1
  BOOLEAN_TO_UINT8_Signals/3(Error) -> Terminator/1

== system Kitchen_Lib/Kitchen/100ms/Kitchn/Subsystem1/Subsystem20 ==
  Kitc_TErrPuls_E2E : Inport
  Terminator40 : Terminator
  Terminator41 : Terminator
  UINT32_Signal : Subsystem  AncestorBlock=E2E_Lib/UINT32_Signal
  wires:
  UINT32_Signal/1(Error) -> Terminator40/1
  UINT32_Signal/2(NotInstalled_NotAvailable) -> Terminator41/1
  Kitc_TErrPuls_E2E/1 -> UINT32_Signal/1(UINT32_SignalIn)

== system Kitchen_Lib/Kitchen/100ms/Kitchn/Subsystem1/Subsystem21 ==
  Kitc_StBuzRe : Inport
  Ground : Ground
  Ground1 : Ground
  SignalE2EStandardBool : Subsystem  AncestorBlock=E2E_Lib/SignalE2EStandardBool
  Kitc_StBuzRe_E2E : Outport
  wires:
  Ground/1 -> SignalE2EStandardBool/2(Error_In)
  Ground1/1 -> SignalE2EStandardBool/3(NotAvailable)
  Kitc_StBuzRe/1 -> SignalE2EStandardBool/1(Sıgnal_In)
  SignalE2EStandardBool/1(Signal_Out) -> Kitc_StBuzRe_E2E/1

== system Kitchen_Lib/Kitchen/100ms/Kitchn/Subsystem1/Subsystem22 ==
  Kitc_StSmlCns : Inport
  Ground : Ground
  Ground1 : Ground
  SignalE2EStandardU16 : Subsystem  AncestorBlock=E2E_Lib/SignalE2EStandardU16
  Kitc_StSmlCns_E2E : Outport
  wires:
  Ground/1 -> SignalE2EStandardU16/2(Error_In)
  Ground1/1 -> SignalE2EStandardU16/3(NotAvailable)
  Kitc_StSmlCns/1 -> SignalE2EStandardU16/1(Sıgnal_In)
  SignalE2EStandardU16/1(Signal_Out) -> Kitc_StSmlCns_E2E/1

== system Kitchen_Lib/Kitchen/100ms/Kitchn/Subsystem1/Subsystem23 ==
  Kitc_StsPwmFreq : Inport
  Ground : Ground
  Ground1 : Ground
  SignalE2EStandardU16 : Subsystem  AncestorBlock=E2E_Lib/SignalE2EStandardU16
  Kitc_StsPwmFreq_E2E : Outport
  wires:
  SignalE2EStandardU16/1(Signal_Out) -> Kitc_StsPwmFreq_E2E/1
  Kitc_StsPwmFreq/1 -> SignalE2EStandardU16/1(Sıgnal_In)
  Ground1/1 -> SignalE2EStandardU16/3(NotAvailable)
  Ground/1 -> SignalE2EStandardU16/2(Error_In)

== system Kitchen_Lib/Kitchen/100ms/Kitchn/Subsystem1/Subsystem24 ==
  Kitc_StTrfr : Inport
  Ground : Ground
  Ground1 : Ground
  SignalE2EStandardBool : Subsystem  AncestorBlock=E2E_Lib/SignalE2EStandardBool
  Kitc_StTrfr_E2E : Outport
  wires:
  SignalE2EStandardBool/1(Signal_Out) -> Kitc_StTrfr_E2E/1
  Kitc_StTrfr/1 -> SignalE2EStandardBool/1(Sıgnal_In)
  Ground1/1 -> SignalE2EStandardBool/3(NotAvailable)
  Ground/1 -> SignalE2EStandardBool/2(Error_In)

== system Kitchen_Lib/Kitchen/100ms/Kitchn/Subsystem1/Subsystem25 ==
  Kitc_StsKitcAcv : Inport
  Ground : Ground
  Ground1 : Ground
  SignalE2EStandardBool : Subsystem  AncestorBlock=E2E_Lib/SignalE2EStandardBool
  Kitc_StsKitcAcv_E2E : Outport
  wires:
  SignalE2EStandardBool/1(Signal_Out) -> Kitc_StsKitcAcv_E2E/1
  Kitc_StsKitcAcv/1 -> SignalE2EStandardBool/1(Sıgnal_In)
  Ground1/1 -> SignalE2EStandardBool/3(NotAvailable)
  Ground/1 -> SignalE2EStandardBool/2(Error_In)

== system Kitchen_Lib/Kitchen/100ms/Kitchn/Subsystem1/Subsystem26 ==
  Kitc_EidWtrTankEmpty : Inport
  Ground : Ground
  Ground1 : Ground
  SignalE2EStandardBool : Subsystem  AncestorBlock=E2E_Lib/SignalE2EStandardBool
  Kitc_EidWtrTankEmpty_E2E : Outport
  wires:
  SignalE2EStandardBool/1(Signal_Out) -> Kitc_EidWtrTankEmpty_E2E/1
  Kitc_EidWtrTankEmpty/1 -> SignalE2EStandardBool/1(Sıgnal_In)
  Ground1/1 -> SignalE2EStandardBool/3(NotAvailable)
  Ground/1 -> SignalE2EStandardBool/2(Error_In)

== system Kitchen_Lib/Kitchen/100ms/Kitchn/Subsystem1/Subsystem27 ==
  Kitc_StRefgtr : Inport
  Ground : Ground
  Ground1 : Ground
  SignalE2EStandardBool : Subsystem  AncestorBlock=E2E_Lib/SignalE2EStandardBool
  Kitc_StRefgtr_E2E : Outport
  wires:
  Ground/1 -> SignalE2EStandardBool/2(Error_In)
  Ground1/1 -> SignalE2EStandardBool/3(NotAvailable)
  Kitc_StRefgtr/1 -> SignalE2EStandardBool/1(Sıgnal_In)
  SignalE2EStandardBool/1(Signal_Out) -> Kitc_StRefgtr_E2E/1

== system Kitchen_Lib/Kitchen/100ms/Kitchn/Subsystem1/Subsystem28 ==
  Kitc_StTrfrInstd : Inport
  Ground : Ground
  Ground1 : Ground
  SignalE2EStandardBool : Subsystem  AncestorBlock=E2E_Lib/SignalE2EStandardBool
  Kitc_StTrfrInstd_E2E : Outport
  wires:
  SignalE2EStandardBool/1(Signal_Out) -> Kitc_StTrfrInstd_E2E/1
  Kitc_StTrfrInstd/1 -> SignalE2EStandardBool/1(Sıgnal_In)
  Ground1/1 -> SignalE2EStandardBool/3(NotAvailable)
  Ground/1 -> SignalE2EStandardBool/2(Error_In)

== system Kitchen_Lib/Kitchen/100ms/Kitchn/Subsystem1/Subsystem29 ==
  LRL_StOverHdLggRiLi : Inport
  Ground : Ground
  Ground1 : Ground
  SignalE2EStandardBool : Subsystem  AncestorBlock=E2E_Lib/SignalE2EStandardBool
  LRL_StOverHdLggRiLi_E2E : Outport
  wires:
  SignalE2EStandardBool/1(Signal_Out) -> LRL_StOverHdLggRiLi_E2E/1
  LRL_StOverHdLggRiLi/1 -> SignalE2EStandardBool/1(Sıgnal_In)
  Ground1/1 -> SignalE2EStandardBool/3(NotAvailable)
  Ground/1 -> SignalE2EStandardBool/2(Error_In)

== system Kitchen_Lib/Kitchen/100ms/Kitchn/Subsystem1/Subsystem3 ==
  Kitc_StHostsCallBlink : Inport
  BOOLEAN_TO_UINT8_Signals : Subsystem  AncestorBlock=E2E_Lib/BOOLEAN_TO_UINT8_Signals
  Logical Operator1 : Logic  Operator=NOT  AllPortsSameDT=off  OutDataTypeStr=boolean
  LogicalOperator25 : Logic  AllPortsSameDT=off  OutDataTypeStr=boolean
  Terminator : Terminator
  Terminator1 : Terminator
  Kitc_StHostsCallBlink_E2E : Outport
  wires:
  Logical Operator1/1 -> LogicalOperator25/1
  LogicalOperator25/1 -> Kitc_StHostsCallBlink_E2E/1
  BOOLEAN_TO_UINT8_Signals/2(Signal|On) -> LogicalOperator25/2
  Kitc_StHostsCallBlink/1 -> BOOLEAN_TO_UINT8_Signals/1(BOOLEAN_TO_UINT8_SignalIn)
  BOOLEAN_TO_UINT8_Signals/4(NotInstalled_NotAvailable) -> Terminator1/1
  BOOLEAN_TO_UINT8_Signals/1(SignalOff) -> Logical Operator1/1
  BOOLEAN_TO_UINT8_Signals/3(Error) -> Terminator/1

== system Kitchen_Lib/Kitchen/100ms/Kitchn/Subsystem1/Subsystem30 ==
  LRL_StOverHdLggRiLi : Inport
  Ground : Ground
  Ground1 : Ground
  SignalE2EStandardBool : Subsystem  AncestorBlock=E2E_Lib/SignalE2EStandardBool
  LRL_StOverHdLggRiLi_E2E : Outport
  wires:
  SignalE2EStandardBool/1(Signal_Out) -> LRL_StOverHdLggRiLi_E2E/1
  LRL_StOverHdLggRiLi/1 -> SignalE2EStandardBool/1(Sıgnal_In)
  Ground1/1 -> SignalE2EStandardBool/3(NotAvailable)
  Ground/1 -> SignalE2EStandardBool/2(Error_In)

== system Kitchen_Lib/Kitchen/100ms/Kitchn/Subsystem1/Subsystem31 ==
  LRL_StOverHdLggRiLi : Inport
  Ground : Ground
  Ground1 : Ground
  SignalE2EStandardBool : Subsystem  AncestorBlock=E2E_Lib/SignalE2EStandardBool
  LRL_StOverHdLggRiLi_E2E : Outport
  wires:
  SignalE2EStandardBool/1(Signal_Out) -> LRL_StOverHdLggRiLi_E2E/1
  LRL_StOverHdLggRiLi/1 -> SignalE2EStandardBool/1(Sıgnal_In)
  Ground1/1 -> SignalE2EStandardBool/3(NotAvailable)
  Ground/1 -> SignalE2EStandardBool/2(Error_In)

== system Kitchen_Lib/Kitchen/100ms/Kitchn/Subsystem1/Subsystem32 ==
  LRL_StOverHdLggRiLi : Inport
  Ground : Ground
  Ground1 : Ground
  SignalE2EStandardBool : Subsystem  AncestorBlock=E2E_Lib/SignalE2EStandardBool
  LRL_StOverHdLggRiLi_E2E : Outport
  wires:
  Ground/1 -> SignalE2EStandardBool/2(Error_In)
  Ground1/1 -> SignalE2EStandardBool/3(NotAvailable)
  LRL_StOverHdLggRiLi/1 -> SignalE2EStandardBool/1(Sıgnal_In)
  SignalE2EStandardBool/1(Signal_Out) -> LRL_StOverHdLggRiLi_E2E/1

== system Kitchen_Lib/Kitchen/100ms/Kitchn/Subsystem1/Subsystem33 ==
  Kitc_StHostsCall : Inport
  Ground : Ground
  Ground1 : Ground
  SignalE2EStandardU16 : Subsystem  AncestorBlock=E2E_Lib/SignalE2EStandardU16
  Kitc_StHostsCall_E2E : Outport
  wires:
  SignalE2EStandardU16/1(Signal_Out) -> Kitc_StHostsCall_E2E/1
  Kitc_StHostsCall/1 -> SignalE2EStandardU16/1(Sıgnal_In)
  Ground1/1 -> SignalE2EStandardU16/3(NotAvailable)
  Ground/1 -> SignalE2EStandardU16/2(Error_In)

== system Kitchen_Lib/Kitchen/100ms/Kitchn/Subsystem1/Subsystem34 ==
  Kitchn_StAcvCode : Inport
  Ground : Ground
  Ground1 : Ground
  SignalE2EStandardU16 : Subsystem  AncestorBlock=E2E_Lib/SignalE2EStandardU16
  Kitchn_StAcvCode_E2E : Outport
  wires:
  SignalE2EStandardU16/1(Signal_Out) -> Kitchn_StAcvCode_E2E/1
  Kitchn_StAcvCode/1 -> SignalE2EStandardU16/1(Sıgnal_In)
  Ground1/1 -> SignalE2EStandardU16/3(NotAvailable)
  Ground/1 -> SignalE2EStandardU16/2(Error_In)

== system Kitchen_Lib/Kitchen/100ms/Kitchn/Subsystem1/Subsystem35 ==
  LRL_StLggRoomRiLi_Frq : Inport
  Ground : Ground
  Ground1 : Ground
  SignalE2EStandardU16 : Subsystem  AncestorBlock=E2E_Lib/SignalE2EStandardU16
  LRL_StLggRoomRiLi_Frq_E2E : Outport
  wires:
  SignalE2EStandardU16/1(Signal_Out) -> LRL_StLggRoomRiLi_Frq_E2E/1
  LRL_StLggRoomRiLi_Frq/1 -> SignalE2EStandardU16/1(Sıgnal_In)
  Ground1/1 -> SignalE2EStandardU16/3(NotAvailable)
  Ground/1 -> SignalE2EStandardU16/2(Error_In)

== system Kitchen_Lib/Kitchen/100ms/Kitchn/Subsystem1/Subsystem36 ==
  CLS_StDoorLockdOutd : Inport
  BOOLEAN_TO_UINT8_Signals : Subsystem  AncestorBlock=E2E_Lib/BOOLEAN_TO_UINT8_Signals
  Logical Operator1 : Logic  Operator=NOT  AllPortsSameDT=off  OutDataTypeStr=boolean
  LogicalOperator25 : Logic  AllPortsSameDT=off  OutDataTypeStr=boolean
  Terminator : Terminator
  Terminator1 : Terminator
  CLS_StDoorLockdOutd_E2E : Outport
  wires:
  Logical Operator1/1 -> LogicalOperator25/1
  BOOLEAN_TO_UINT8_Signals/3(Error) -> Terminator/1
  BOOLEAN_TO_UINT8_Signals/1(SignalOff) -> Logical Operator1/1
  BOOLEAN_TO_UINT8_Signals/4(NotInstalled_NotAvailable) -> Terminator1/1
  CLS_StDoorLockdOutd/1 -> BOOLEAN_TO_UINT8_Signals/1(BOOLEAN_TO_UINT8_SignalIn)
  BOOLEAN_TO_UINT8_Signals/2(Signal|On) -> LogicalOperator25/2
  LogicalOperator25/1 -> CLS_StDoorLockdOutd_E2E/1

== system Kitchen_Lib/Kitchen/100ms/Kitchn/Subsystem1/Subsystem4 ==
  Kitc_StHostsCallBlinkUpprDeck : Inport
  BOOLEAN_TO_UINT8_Signals : Subsystem  AncestorBlock=E2E_Lib/BOOLEAN_TO_UINT8_Signals
  Logical Operator1 : Logic  Operator=NOT  AllPortsSameDT=off  OutDataTypeStr=boolean
  LogicalOperator25 : Logic  AllPortsSameDT=off  OutDataTypeStr=boolean
  Terminator : Terminator
  Terminator1 : Terminator
  Kitc_StHostsCallBlinkUpprDeck_E2E : Outport
  wires:
  Logical Operator1/1 -> LogicalOperator25/1
  BOOLEAN_TO_UINT8_Signals/3(Error) -> Terminator/1
  BOOLEAN_TO_UINT8_Signals/1(SignalOff) -> Logical Operator1/1
  BOOLEAN_TO_UINT8_Signals/4(NotInstalled_NotAvailable) -> Terminator1/1
  Kitc_StHostsCallBlinkUpprDeck/1 -> BOOLEAN_TO_UINT8_Signals/1(BOOLEAN_TO_UINT8_SignalIn)
  BOOLEAN_TO_UINT8_Signals/2(Signal|On) -> LogicalOperator25/2
  LogicalOperator25/1 -> Kitc_StHostsCallBlinkUpprDeck_E2E/1

== system Kitchen_Lib/Kitchen/100ms/Kitchn/Subsystem1/Subsystem41 ==
  Kitc_StLrgCns : Inport
  Ground : Ground
  Ground1 : Ground
  SignalE2EStandardU16 : Subsystem  AncestorBlock=E2E_Lib/SignalE2EStandardU16
  Kitc_StLrgCns_E2E : Outport
  wires:
  SignalE2EStandardU16/1(Signal_Out) -> Kitc_StLrgCns_E2E/1
  Kitc_StLrgCns/1 -> SignalE2EStandardU16/1(Sıgnal_In)
  Ground1/1 -> SignalE2EStandardU16/3(NotAvailable)
  Ground/1 -> SignalE2EStandardU16/2(Error_In)

== system Kitchen_Lib/Kitchen/100ms/Kitchn/Subsystem1/Subsystem5 ==
  GW_StUvLoPrio : Inport
  BOOLEAN_TO_UINT8_Signals : Subsystem  AncestorBlock=E2E_Lib/BOOLEAN_TO_UINT8_Signals
  Logical Operator : Logic  AllPortsSameDT=off  OutDataTypeStr=boolean
  Logical Operator1 : Logic  Operator=NOT  AllPortsSameDT=off  OutDataTypeStr=boolean
  Terminator : Terminator
  Terminator1 : Terminator
  GW_StUvLoPrio_E2E : Outport
  wires:
  BOOLEAN_TO_UINT8_Signals/1(SignalOff) -> Logical Operator1/1
  Logical Operator/1 -> GW_StUvLoPrio_E2E/1
  GW_StUvLoPrio/1 -> BOOLEAN_TO_UINT8_Signals/1(BOOLEAN_TO_UINT8_SignalIn)
  Logical Operator1/1 -> Logical Operator/1
  BOOLEAN_TO_UINT8_Signals/3(Error) -> Terminator/1
  BOOLEAN_TO_UINT8_Signals/4(NotInstalled_NotAvailable) -> Terminator1/1
  BOOLEAN_TO_UINT8_Signals/2(Signal|On) -> Logical Operator/2

== system Kitchen_Lib/Kitchen/100ms/Kitchn/Subsystem1/Subsystem6 ==
  Kitc_StsWtrTankEmpty : Inport
  BOOLEAN_TO_UINT8_Signals : Subsystem  AncestorBlock=E2E_Lib/BOOLEAN_TO_UINT8_Signals
  Logical Operator1 : Logic  Operator=NOT  AllPortsSameDT=off  OutDataTypeStr=boolean
  LogicalOperator25 : Logic  AllPortsSameDT=off  OutDataTypeStr=boolean
  Terminator : Terminator
  Terminator1 : Terminator
  Kitc_StsWtrTankEmpty_E2E : Outport
  wires:
  Logical Operator1/1 -> LogicalOperator25/1
  LogicalOperator25/1 -> Kitc_StsWtrTankEmpty_E2E/1
  BOOLEAN_TO_UINT8_Signals/2(Signal|On) -> LogicalOperator25/2
  Kitc_StsWtrTankEmpty/1 -> BOOLEAN_TO_UINT8_Signals/1(BOOLEAN_TO_UINT8_SignalIn)
  BOOLEAN_TO_UINT8_Signals/4(NotInstalled_NotAvailable) -> Terminator1/1
  BOOLEAN_TO_UINT8_Signals/1(SignalOff) -> Logical Operator1/1
  BOOLEAN_TO_UINT8_Signals/3(Error) -> Terminator/1

== system Kitchen_Lib/Kitchen/100ms/Kitchn/Subsystem1/Subsystem7 ==
  GW_StClmp50Off3Sec : Inport
  BOOLEAN_TO_UINT8_Signals : Subsystem  AncestorBlock=E2E_Lib/BOOLEAN_TO_UINT8_Signals
  Logical Operator : Logic  AllPortsSameDT=off  OutDataTypeStr=boolean
  Logical Operator1 : Logic  Operator=NOT  AllPortsSameDT=off  OutDataTypeStr=boolean
  Terminator : Terminator
  Terminator1 : Terminator
  GW_StClmp50Off3Sec_E2E : Outport
  wires:
  BOOLEAN_TO_UINT8_Signals/1(SignalOff) -> Logical Operator1/1
  Logical Operator/1 -> GW_StClmp50Off3Sec_E2E/1
  GW_StClmp50Off3Sec/1 -> BOOLEAN_TO_UINT8_Signals/1(BOOLEAN_TO_UINT8_SignalIn)
  Logical Operator1/1 -> Logical Operator/1
  BOOLEAN_TO_UINT8_Signals/3(Error) -> Terminator/1
  BOOLEAN_TO_UINT8_Signals/4(NotInstalled_NotAvailable) -> Terminator1/1
  BOOLEAN_TO_UINT8_Signals/2(Signal|On) -> Logical Operator/2

== system Kitchen_Lib/Kitchen/100ms/Kitchn/Subsystem1/Subsystem8 ==
  Kitc_StsHostsCallAcvUpprDeck : Inport
  BOOLEAN_TO_UINT8_Signals : Subsystem  AncestorBlock=E2E_Lib/BOOLEAN_TO_UINT8_Signals
  Logical Operator1 : Logic  Operator=NOT  AllPortsSameDT=off  OutDataTypeStr=boolean
  LogicalOperator25 : Logic  AllPortsSameDT=off  OutDataTypeStr=boolean
  Terminator : Terminator
  Terminator1 : Terminator
  Kitc_StsHostsCallAcvUpprDeck_E2E : Outport
  wires:
  Logical Operator1/1 -> LogicalOperator25/1
  BOOLEAN_TO_UINT8_Signals/3(Error) -> Terminator/1
  BOOLEAN_TO_UINT8_Signals/1(SignalOff) -> Logical Operator1/1
  BOOLEAN_TO_UINT8_Signals/4(NotInstalled_NotAvailable) -> Terminator1/1
  Kitc_StsHostsCallAcvUpprDeck/1 -> BOOLEAN_TO_UINT8_Signals/1(BOOLEAN_TO_UINT8_SignalIn)
  BOOLEAN_TO_UINT8_Signals/2(Signal|On) -> LogicalOperator25/2
  LogicalOperator25/1 -> Kitc_StsHostsCallAcvUpprDeck_E2E/1

== system Kitchen_Lib/Kitchen/100ms/Kitchn/Subsystem1/Subsystem9 ==
  Kitc_StTrfrWoutNewStrt : Inport
  BOOLEAN_TO_UINT8_Signals : Subsystem  AncestorBlock=E2E_Lib/BOOLEAN_TO_UINT8_Signals
  Logical Operator : Logic  AllPortsSameDT=off  OutDataTypeStr=boolean
  Logical Operator1 : Logic  Operator=NOT  AllPortsSameDT=off  OutDataTypeStr=boolean
  Terminator : Terminator
  Terminator1 : Terminator
  Kitc_StTrfrWoutNewStrt_E2E : Outport
  wires:
  BOOLEAN_TO_UINT8_Signals/2(Signal|On) -> Logical Operator/2
  BOOLEAN_TO_UINT8_Signals/4(NotInstalled_NotAvailable) -> Terminator1/1
  BOOLEAN_TO_UINT8_Signals/3(Error) -> Terminator/1
  Logical Operator1/1 -> Logical Operator/1
  Kitc_StTrfrWoutNewStrt/1 -> BOOLEAN_TO_UINT8_Signals/1(BOOLEAN_TO_UINT8_SignalIn)
  Logical Operator/1 -> Kitc_StTrfrWoutNewStrt_E2E/1
  BOOLEAN_TO_UINT8_Signals/1(SignalOff) -> Logical Operator1/1

== system Kitchen_Lib/Kitchen/100ms/Kitchn/Subsystem1/Subsystem1/BOOLEAN_TO_UINT8_Signals ==
  BOOLEAN_TO_UINT8_SignalIn : Inport
  Constant : Constant  Value=uint8(0)
  Constant1 : Constant  Value=uint8(1)
  Constant2 : Constant  Value=uint8(2)
  Constant3 : Constant  Value=uint8(3)
  Data Type Conversion : DataTypeConversion  OutDataTypeStr=uint8  SaturateOnIntegerOverflow=off  RndMeth=Floor
  Relational Operator{,1..3} (4 alike) : RelationalOperator  Operator===  OutDataTypeStr=boolean  InputSameDT=off
  SignalOff : Outport
  Signal|On : Outport  Port=2
  Error : Outport  Port=3
  NotInstalled_NotAvailable : Outport  Port=4
  wires:
  Relational Operator3/1 -> NotInstalled_NotAvailable/1
  Relational Operator2/1 -> Error/1
  Relational Operator1/1 -> Signal|On/1
  Relational Operator/1 -> SignalOff/1
  Data Type Conversion/1 -> Relational Operator/1, Relational Operator2/1, Relational Operator3/1, Relational Operator1/1
  Constant2/1 -> Relational Operator2/2
  Constant/1 -> Relational Operator/2
  BOOLEAN_TO_UINT8_SignalIn/1 -> Data Type Conversion/1
  Constant3/1 -> Relational Operator3/2
  Constant1/1 -> Relational Operator1/2

== system Kitchen_Lib/Kitchen/100ms/Kitchn/Subsystem1/Subsystem10/UINT8_Signal ==
  UINT8_SignalIn : Inport
  Constant : Constant  Value=uint8(0)
  Constant1 : Constant  Value=uint8(1)
  Constant2 : Constant  Value=uint8(254)
  Constant3 : Constant  Value=uint8(255)
  Data Type Conversion : DataTypeConversion  OutDataTypeStr=uint8  SaturateOnIntegerOverflow=off  RndMeth=Floor
  Relational Operator{,1..3} (4 alike) : RelationalOperator  Operator===  OutDataTypeStr=boolean  InputSameDT=off
  Terminator : Terminator
  Terminator1 : Terminator
  Error : Outport
  NotInstalled_NotAvailable : Outport  Port=2
  wires:
  Constant1/1 -> Relational Operator1/2
  Constant3/1 -> Relational Operator3/2
  UINT8_SignalIn/1 -> Data Type Conversion/1
  Constant/1 -> Relational Operator/2
  Constant2/1 -> Relational Operator2/2
  Data Type Conversion/1 -> Relational Operator1/1, Relational Operator3/1, Relational Operator2/1, Relational Operator/1
  Relational Operator2/1 -> Error/1
  Relational Operator3/1 -> NotInstalled_NotAvailable/1
  Relational Operator/1 -> Terminator/1
  Relational Operator1/1 -> Terminator1/1

== system Kitchen_Lib/Kitchen/100ms/Kitchn/Subsystem1/Subsystem11/UINT8_Signal ==
  UINT8_SignalIn : Inport
  Constant : Constant  Value=uint8(0)
  Constant1 : Constant  Value=uint8(1)
  Constant2 : Constant  Value=uint8(254)
  Constant3 : Constant  Value=uint8(255)
  Data Type Conversion : DataTypeConversion  OutDataTypeStr=uint8  SaturateOnIntegerOverflow=off  RndMeth=Floor
  Relational Operator{,1..3} (4 alike) : RelationalOperator  Operator===  OutDataTypeStr=boolean  InputSameDT=off
  Terminator : Terminator
  Terminator1 : Terminator
  Error : Outport
  NotInstalled_NotAvailable : Outport  Port=2
  wires:
  Constant1/1 -> Relational Operator1/2
  Constant3/1 -> Relational Operator3/2
  UINT8_SignalIn/1 -> Data Type Conversion/1
  Constant/1 -> Relational Operator/2
  Constant2/1 -> Relational Operator2/2
  Data Type Conversion/1 -> Relational Operator1/1, Relational Operator3/1, Relational Operator2/1, Relational Operator/1
  Relational Operator2/1 -> Error/1
  Relational Operator3/1 -> NotInstalled_NotAvailable/1
  Relational Operator/1 -> Terminator/1
  Relational Operator1/1 -> Terminator1/1

== system Kitchen_Lib/Kitchen/100ms/Kitchn/Subsystem1/Subsystem12/BOOLEAN_TO_UINT8_Signals ==
  BOOLEAN_TO_UINT8_SignalIn : Inport
  Constant : Constant  Value=uint8(0)
  Constant1 : Constant  Value=uint8(1)
  Constant2 : Constant  Value=uint8(2)
  Constant3 : Constant  Value=uint8(3)
  Data Type Conversion : DataTypeConversion  OutDataTypeStr=uint8  SaturateOnIntegerOverflow=off  RndMeth=Floor
  Relational Operator{,1..3} (4 alike) : RelationalOperator  Operator===  OutDataTypeStr=boolean  InputSameDT=off
  SignalOff : Outport
  Signal|On : Outport  Port=2
  Error : Outport  Port=3
  NotInstalled_NotAvailable : Outport  Port=4
  wires:
  Relational Operator3/1 -> NotInstalled_NotAvailable/1
  Relational Operator2/1 -> Error/1
  Relational Operator1/1 -> Signal|On/1
  Relational Operator/1 -> SignalOff/1
  Data Type Conversion/1 -> Relational Operator/1, Relational Operator2/1, Relational Operator3/1, Relational Operator1/1
  Constant2/1 -> Relational Operator2/2
  Constant/1 -> Relational Operator/2
  BOOLEAN_TO_UINT8_SignalIn/1 -> Data Type Conversion/1
  Constant3/1 -> Relational Operator3/2
  Constant1/1 -> Relational Operator1/2

== system Kitchen_Lib/Kitchen/100ms/Kitchn/Subsystem1/Subsystem13/BOOLEAN_TO_UINT8_Signals ==
  BOOLEAN_TO_UINT8_SignalIn : Inport
  Constant : Constant  Value=uint8(0)
  Constant1 : Constant  Value=uint8(1)
  Constant2 : Constant  Value=uint8(2)
  Constant3 : Constant  Value=uint8(3)
  Data Type Conversion : DataTypeConversion  OutDataTypeStr=uint8  SaturateOnIntegerOverflow=off  RndMeth=Floor
  Relational Operator{,1..3} (4 alike) : RelationalOperator  Operator===  OutDataTypeStr=boolean  InputSameDT=off
  SignalOff : Outport
  Signal|On : Outport  Port=2
  Error : Outport  Port=3
  NotInstalled_NotAvailable : Outport  Port=4
  wires:
  Relational Operator3/1 -> NotInstalled_NotAvailable/1
  Relational Operator2/1 -> Error/1
  Relational Operator1/1 -> Signal|On/1
  Relational Operator/1 -> SignalOff/1
  Data Type Conversion/1 -> Relational Operator/1, Relational Operator2/1, Relational Operator3/1, Relational Operator1/1
  Constant2/1 -> Relational Operator2/2
  Constant/1 -> Relational Operator/2
  BOOLEAN_TO_UINT8_SignalIn/1 -> Data Type Conversion/1
  Constant3/1 -> Relational Operator3/2
  Constant1/1 -> Relational Operator1/2

== system Kitchen_Lib/Kitchen/100ms/Kitchn/Subsystem1/Subsystem14/BOOLEAN_TO_UINT8_Signals ==
  BOOLEAN_TO_UINT8_SignalIn : Inport
  Constant : Constant  Value=uint8(0)
  Constant1 : Constant  Value=uint8(1)
  Constant2 : Constant  Value=uint8(2)
  Constant3 : Constant  Value=uint8(3)
  Data Type Conversion : DataTypeConversion  OutDataTypeStr=uint8  SaturateOnIntegerOverflow=off  RndMeth=Floor
  Relational Operator{,1..3} (4 alike) : RelationalOperator  Operator===  OutDataTypeStr=boolean  InputSameDT=off
  SignalOff : Outport
  Signal|On : Outport  Port=2
  Error : Outport  Port=3
  NotInstalled_NotAvailable : Outport  Port=4
  wires:
  Relational Operator3/1 -> NotInstalled_NotAvailable/1
  Relational Operator2/1 -> Error/1
  Relational Operator1/1 -> Signal|On/1
  Relational Operator/1 -> SignalOff/1
  Data Type Conversion/1 -> Relational Operator/1, Relational Operator2/1, Relational Operator3/1, Relational Operator1/1
  Constant2/1 -> Relational Operator2/2
  Constant/1 -> Relational Operator/2
  BOOLEAN_TO_UINT8_SignalIn/1 -> Data Type Conversion/1
  Constant3/1 -> Relational Operator3/2
  Constant1/1 -> Relational Operator1/2

== system Kitchen_Lib/Kitchen/100ms/Kitchn/Subsystem1/Subsystem15/BOOLEAN_TO_UINT8_Signals ==
  BOOLEAN_TO_UINT8_SignalIn : Inport
  Constant : Constant  Value=uint8(0)
  Constant1 : Constant  Value=uint8(1)
  Constant2 : Constant  Value=uint8(2)
  Constant3 : Constant  Value=uint8(3)
  Data Type Conversion : DataTypeConversion  OutDataTypeStr=uint8  SaturateOnIntegerOverflow=off  RndMeth=Floor
  Relational Operator{,1..3} (4 alike) : RelationalOperator  Operator===  OutDataTypeStr=boolean  InputSameDT=off
  SignalOff : Outport
  Signal|On : Outport  Port=2
  Error : Outport  Port=3
  NotInstalled_NotAvailable : Outport  Port=4
  wires:
  Relational Operator3/1 -> NotInstalled_NotAvailable/1
  Relational Operator2/1 -> Error/1
  Relational Operator1/1 -> Signal|On/1
  Relational Operator/1 -> SignalOff/1
  Data Type Conversion/1 -> Relational Operator/1, Relational Operator2/1, Relational Operator3/1, Relational Operator1/1
  Constant2/1 -> Relational Operator2/2
  Constant/1 -> Relational Operator/2
  BOOLEAN_TO_UINT8_SignalIn/1 -> Data Type Conversion/1
  Constant3/1 -> Relational Operator3/2
  Constant1/1 -> Relational Operator1/2
